simulink model "FDI_sbox_ttime"  (R2018a)
settings: Solver=ode45  StartTime=0.0  StopTime=.4  MaxStep=1e-4  RelTol=1e-3
InitFcn:
  | SimulinkInit
values from neighbouring files (symbols this model uses):
  ssAl = [-2.49999998232 0 0 0 376.789751319 0 -3.33333337039 0 0 376.789751319 0 0 ... (25 elements, 5x5)]    [modeloElectrico.mat]
  ssBl = [24.9999999997 0 0 0 0 0 33.333333333 0 0 0 0 0 ... (15 elements, 5x3)]    [modeloElectrico.mat]
  ssCl = [-0.229841748304 -0.00828937452901 0.991710625471 0 -0.229841748304 0.991710625471 -0.00828937452901 0 0.770158251696 -0.00828937452901 -0.00828937452901 0 ... (20 elements, 4x5)]    [modeloElectrico.mat]
undefined symbols (not defined in the file or in its folder): J, K1, K2, K3, P, Tao1, Tao2
libraries: powerlib x25, truetime x11, dsparch4 x5, mpclib x2, simulink x1, powerlib_meascontrol x1
settings Model: Creator=cmparedes  LastModifiedBy=erich

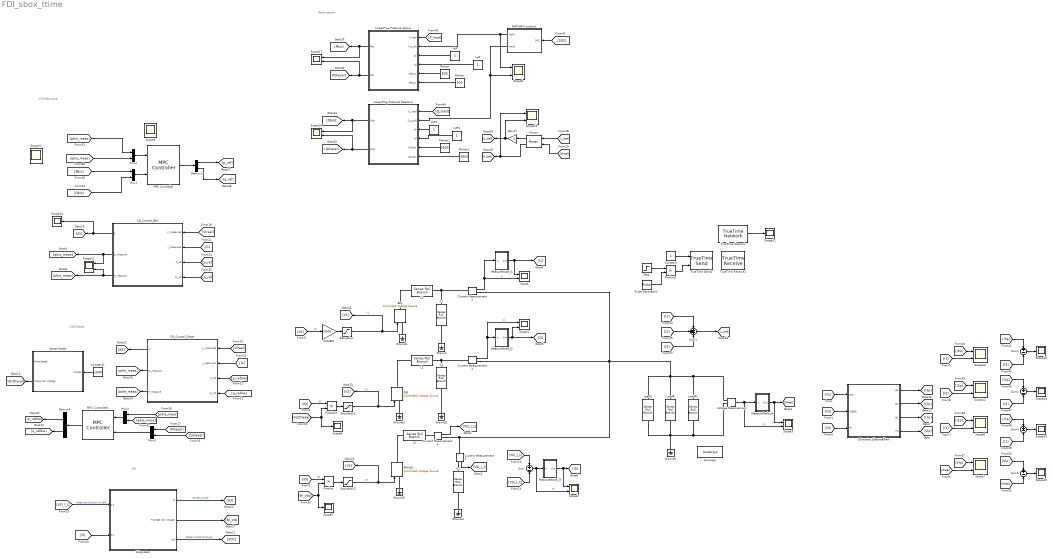
== system FDI_sbox_ttime ==
  note: Optimizacion
  note: CSI2-Diesel
  note: VSI
  note: CSI1-Biomasa
  2VdcBIO : Gain  Gain=2*500
  BIO : powerlib/Electrical Sources/Controlled Voltage Source  Initialize=on  Source_Type=DC  Amplitude=0  Phase=0  Frequency=0  Measurements=None
  C1 : powerlib/Elements/Series RLC Branch  LConnTagsString=__new0  RConnTagsString=__new0  BranchType=C  Resistance=1  Inductance=1e-3  SetiL0=off  InitialCurrent=0  Capacitance=22e-6  Setx0=off  InitialVoltage=0  Measurements=None
  C2 : powerlib/Elements/Series RLC Branch  LConnTagsString=__new0  RConnTagsString=__new0  BranchType=C  Resistance=1  Inductance=1e-3  SetiL0=off  InitialCurrent=0  Capacitance=22e-6  Setx0=off  InitialVoltage=0  Measurements=None
  C3 : powerlib/Elements/Series RLC Branch  LConnTagsString=__new0  RConnTagsString=__new0  BranchType=C  Resistance=1  Inductance=1e-3  SetiL0=off  InitialCurrent=0  Capacitance=610e-6  Setx0=off  InitialVoltage=0  Measurements=None
  CSI_Control_BIO : Subsystem  mask{A=[0.0201   -0.039932     0.01986], B=[1     -1.9966       0.998], T=0.0001, st_time=.1, Dn=[1     -1.0364], Dd=[1    -0.96364]}
      mask prompts: A "Numerador del control PR(z)"; B "Denominador del control PR(z)"; T "Tiempo de muestreo"; st_time "Tiempo_muerto"; Dn "Dn (Numerador de D(z))"; Dd "Dd (numerador de D(z))"
      mask DialogControl descripcion Prompt: Lazo de control de corriente para inversor monofasico. La entrada es un setpoint de potencia [P, Q]. Con ese setpoint se calcula la referencia de corriente sinusoidal deacuerdo a la tension medida de la red. Por lo anterior este controlador solo es valido para un inversor conectado a la red pues hara que se comporte como un CSI.
      mask DialogControl Control2 Prompt: Dn y Dd corresponden al numerador y denominador de la funcion de transferencia en Z (denominada D(z)) que hara un desfase de 90 de las señales medidas de tension y corriente del inversor. Estos desfases permiten mimificar las señales alfa y beta, de esta forma usar la misma teoria de potencia instantanea para el caso monofasico.
  CSI_Control_Diesel : Subsystem  mask{A=[0.0201   -0.039932     0.01986], B=[1     -1.9966       0.998], T=0.0001, st_time=.1, Dn=[1     -1.0364], Dd=[1    -0.96364]}
      mask prompts: A "Numerador del control PR(z)"; B "Denominador del control PR(z)"; T "Tiempo de muestreo"; st_time "Tiempo_muerto"; Dn "Dn (Numerador de D(z))"; Dd "Dd (numerador de D(z))"
      mask DialogControl descripcion Prompt: Lazo de control de corriente para inversor monofasico. La entrada es un setpoint de potencia [P, Q]. Con ese setpoint se calcula la referencia de corriente sinusoidal deacuerdo a la tension medida de la red. Por lo anterior este controlador solo es valido para un inversor conectado a la red pues hara que se comporte como un CSI.
      mask DialogControl Control2 Prompt: Dn y Dd corresponden al numerador y denominador de la funcion de transferencia en Z (denominada D(z)) que hara un desfase de 90 de las señales medidas de tension y corriente del inversor. Estos desfases permiten mimificar las señales alfa y beta, de esta forma usar la misma teoria de potencia instantanea para el caso monofasico.
  Constant : Constant
  Constant1 : Constant  Value=1000
  Current Measurement{1..4} (4 alike) : powerlib/Measurements/Current Measurement  PhasorSimulation=off  OutputType=Complex  PSBequivalent=0
  DIE : powerlib/Electrical Sources/Controlled Voltage Source  Initialize=on  Source_Type=DC  Amplitude=0  Phase=0  Frequency=0  Measurements=None
  Demux1 : Demux  Outputs=2
  Demux4 : Demux  Outputs=2
  Diesel Model : Subsystem
  Gain17 : Gain  Gain=-1
  Ground{,1..6} (7 alike) : powerlib/Elements/Ground  LConnTagsString=a
  L1 : powerlib/Elements/Series RLC Branch  LConnTagsString=__new0  RConnTagsString=__new0  BranchType=RL  Resistance=.1  Inductance=40e-3  SetiL0=off  InitialCurrent=0  Capacitance=1e-6  Setx0=off  InitialVoltage=0  Measurements=None
  L2 : powerlib/Elements/Series RLC Branch  LConnTagsString=__new0  RConnTagsString=__new0  BranchType=RL  Resistance=.1  Inductance=30e-3  SetiL0=off  InitialCurrent=0  Capacitance=1e-6  Setx0=off  InitialVoltage=0  Measurements=None
  L3 : powerlib/Elements/Series RLC Branch  LConnTagsString=__new0  RConnTagsString=__new0  BranchType=RL  Resistance=1e-3  Inductance=5e-3  SetiL0=off  InitialCurrent=0  Capacitance=1e-6  Setx0=off  InitialVoltage=0  Measurements=None
  LinearProg Potencia Activa : MATLAB Function  TreatAsAtomicUnit=on  SystemSampleTime=.03
  LinearProg Potenica Reactiva : MATLAB Function  TreatAsAtomicUnit=on  SystemSampleTime=.03
  LoadC : powerlib/Elements/Series RLC Branch  LConnTagsString=__new0  RConnTagsString=__new0  BranchType=C  Resistance=1  Inductance=1e-3  SetiL0=off  InitialCurrent=0  Capacitance=2000e-6  Setx0=off  InitialVoltage=0  Measurements=None
  LoadR : powerlib/Elements/Series RLC Branch  LConnTagsString=__new0  RConnTagsString=__new0  BranchType=R  Resistance=10  Inductance=1e-3  SetiL0=off  InitialCurrent=0  Capacitance=1e-6  Setx0=off  InitialVoltage=0  Measurements=None
  LoadRL : powerlib/Elements/Series RLC Branch  LConnTagsString=__new0  RConnTagsString=__new0  BranchType=RL  Resistance=10  Inductance=5.2  SetiL0=off  InitialCurrent=0  Capacitance=1e-6  Setx0=off  InitialVoltage=0  Measurements=None
  MATLAB Function1 : MATLAB Function  TreatAsAtomicUnit=on
  MPC Controller : mpclib/MPC Controller  mpcobj=mpcobj  x0=[]  is_multiple=0  enable_value=0  return_u0=off  updateMPCinCallerWorkspace=on  ref_from_ws=off  ref_signal_name=[]  ref_preview=on  md_from_ws=off  md_signal_name=[]  md_preview=on  from_project=off  project_file=MPCtask.mat  md_inport=off  mv_inport=off  cost_outport=off  return_sequence=off  return_qpstatus=off  return_state=off  state_inport=off  lims_inport=off  cc_inport=off  ywt_inport=off  is_designfromscratch=0  uwt_inport=off  duwt_inport=off  rhoeps_inport=off  uref_inport=off  n_ts=0.1  n_p=100  n_mv=2  n_md=0  n_ud=0  n_mo=2  n_uo=0  BlockDataType=double  SampleTimeInherited=off  switch_inport=off
  MPC Controller1 : mpclib/MPC Controller  mpcobj=mpcobj  x0=[]  is_multiple=0  enable_value=0  return_u0=off  updateMPCinCallerWorkspace=on  ref_from_ws=off  ref_signal_name=[]  ref_preview=on  md_from_ws=off  md_signal_name=[]  md_preview=on  from_project=off  project_file=MPCtask.mat  md_inport=off  mv_inport=off  cost_outport=off  return_sequence=off  return_qpstatus=off  return_state=off  state_inport=off  lims_inport=off  cc_inport=off  ywt_inport=off  is_designfromscratch=0  uwt_inport=off  duwt_inport=off  rhoeps_inport=off  uref_inport=off  n_ts=0.1  n_p=100  n_mv=2  n_md=0  n_ud=0  n_mo=2  n_uo=0  BlockDataType=double  SampleTimeInherited=off  switch_inport=off
  MeasureNode_I1 : Subsystem
  MeasureNode_I2 : Subsystem
  MeasureNode_I3 : Subsystem
  MeasureNode_I4 : Subsystem
  Mux{1..4} (4 alike) : Mux  Inputs=2
  PH(VSI) : powerlib/Electrical Sources/Controlled Voltage Source  Initialize=on  Source_Type=DC  Amplitude=0  Phase=0  Frequency=0  Measurements=None
  Pbmax : Constant  Value=500
  Pbmax1 : Constant  Value=3500
  Pdmax : Constant  Value=500
  Pdmax1 : Constant  Value=3500
  Power : powerlib_meascontrol/Measurements/Power  Freq=60  Vinit=[1, 0]  Iinit=[1, 0]  Ts=0
      settings: SourceProductName=Simscape Power Systems
  Product : Product
  Product1 : Product
  Product2 : Product
  Pulse Generator1 : DiscretePulseGenerator  PulseType=Time based  Period=1e-4  PulseWidth=5
  SSversion_ElectricalPart : Subsystem
  Saturation : Saturate  UpperLimit=500  LowerLimit=-500
  Saturation1 : Saturate  UpperLimit=500  LowerLimit=-500
  Saturation2 : Saturate  UpperLimit=500  LowerLimit=-500
  Scope{,1..3,6..13,16..17,21} (15 alike) : Scope  NumInputPorts=2
  Scope{4..5,14..15,18..20,22} (8 alike) : Scope
  Step : Step  Time=5  SampleTime=0
  Subsystem : Subsystem
  Sum{,2..5} (5 alike) : Sum  Inputs=+-
  Sum1 : Sum  Inputs=+++
  TrueTime Network : truetime/TrueTime Network  nwtype=CSMA/CD (Ethernet)  nwnbr=1  nnodes=10  rate=100000000000  minsize=512  lossprob=0  seed=0  bandwidths=[0.5 0.5]  slotsize=512  schedule=[1 1 2]  memsize=80000  buftype=Common buffer  overflow=Retransmit  dynSchedule=0  miniSlotSize=0  NIT=0  QSortMode=FIFO  sync=0  irtSchedule=0  nrtLength=0  nodeGraph=0  scheduleoutput=on
  TrueTime Receive1 : truetime/TrueTime Receive  nwnbr=1  receiver=10  outdim=1  triggeroutput=on  senderoutput=off  lengthoutput=off  priorityoutput=off  timestampoutput=off  signalpoweroutput=off  msgIDoutput=off
  TrueTime Send1 : truetime/TrueTime Send  trigger=falling  nwnbr=1  sender=9  indim=1  recsource=internal  receiver=10  lengthsource=internal  length=70000000  priosource=internal  prio=1  msgIDsource=internal  msgID=0  dynamicSegment=dynamic
  Voltage Measurement : powerlib/Measurements/Voltage Measurement  PhasorSimulation=off  OutputType=Complex  PSBequivalent=0
  kbP : Constant
  kbP1 : Constant
  kdP : Constant
  kdP1 : Constant
  powergui : powerlib/powergui  Priority=1  SimulationMode=Continuous  SampleTime=50e-6  frequency=60  Iterations=50  frequencyindice=0  Pbase=100e6  ErrMax=1e-4  UnitsV=kV  UnitsW=MW  buscounter=0  FunctionMessages=off  echomessages=off  EnableUseOfTLC=off  CurrentSourceSwitches=off  DisableSnubberDevices=off  DisableRonSwitches=off  DisableVfSwitches=off  DisplayEquations=off  SolverType=Tustin/Backward Euler (TBE)  Interpol=off  ExternalGateDelay=off  methode=off  Ts=100  x0status=blocks  SPID=on  SwTol=0  HookPort=off  RestoreLinks=warning  ResistiveCurrentMeasurement=off  Frange=[0:2:500]  Ylog=off  Xlog=on  ShowGrid=off  save=off  variable=ZData  structure=0  ZoomFFT=off  StartTime=0.0  cycles=1  DisplayStyle=1  fundamental=60  FreqAxis=off  MaxFrequency=1000  frequencyindicesteady=1  RmsSteady=1  display=off
  wires:
  [d1] -> 2VdcBIO/1  "d1"
  [d2] -> Product1/1  "d2"
  [d3] -> Product/1  "d3"
  Current Measurement2/1 -> MeasureNode_I1/1(in), Scope/2  "I1"
  Current Measurement1/1 -> Scope1/1, MeasureNode_I2/1(in)  "I2"
  Sum/1 -> MeasureNode_I3/1(in), Scope2/2  "I3"
  Voltage Measurement/1 -> Scope3/2, MeasureNode_I4/1(in)  "VL"
  Pdmax1/1 -> LinearProg Potenica Reactiva/5(QdMax)
  [Pbio] -> Mux1/1
  Mux1/1 -> MPC Controller/2
  [SOC] -> MATLAB Function1/1(SOC)
  [Qbio] -> Mux1/2
  [Qdiesel] -> Mux3/2
  [qdie_meas] -> Mux4/2
  [p_refdie] -> CSI_Control_Diesel/3(P_ref)
  [Pdiesel] -> Mux3/1
  [Q_load] -> LinearProg Potenica Reactiva/1(Q_load)
  CSI_Control_BIO/2(Q_measure) -> [qbio_meas], Scope21/1
  [qbio_meas] -> Mux2/2
  Pbmax1/1 -> LinearProg Potenica Reactiva/6(QbMax)
  [q_refdie] -> CSI_Control_Diesel/4(Q_ref)
  LinearProg Potencia Activa/1(Pbo) -> Scope17/1, [Pbio]
  kdP1/1 -> LinearProg Potenica Reactiva/4(kd)
  MATLAB Function1/2(MaxQ) -> Scope9/2, LinearProg Potenica Reactiva/2(Q_e_alt)
  CSI_Control_BIO/1(D) -> [d1], Scope14/1
  Demux1/2 -> [q_ref]
  Pdmax/1 -> LinearProg Potencia Activa/5(PdMax)
  Pbmax/1 -> LinearProg Potencia Activa/6(PbMax)
  [P_load] -> LinearProg Potencia Activa/1(P_load)
  Demux4/2 -> [q_refdie]
  kbP/1 -> LinearProg Potencia Activa/3(kb)
  Mux4/1 -> MPC Controller1/1
  Demux1/1 -> [p_ref]
  kbP1/1 -> LinearProg Potenica Reactiva/3(kb)
  LinearProg Potenica Reactiva/1(Qbo) -> Scope16/1, [Qbio]
  MPC Controller/1 -> Demux1/1
  [pdie_meas] -> Mux4/1
  LinearProg Potenica Reactiva/2(Qdo) -> Scope16/2, [Qdiesel]
  Mux3/1 -> MPC Controller1/2
  Demux4/1 -> [p_refdie]
  CSI_Control_Diesel/2(Q_measure) -> [qdie_meas]
  Mux2/1 -> MPC Controller/1
  [q_ref] -> CSI_Control_BIO/4(Q_ref)
  CSI_Control_BIO/3(P_measure) -> Scope21/2, [pbio_meas]
  CSI_Control_Diesel/3(P_measure) -> [pdie_meas]
  [Vlreal] -> CSI_Control_BIO/1(V_measured)
  MPC Controller1/1 -> Demux4/1
  LinearProg Potencia Activa/2(Pdo) -> Scope17/2, [Pdiesel]
  MATLAB Function1/1(MaxP) -> Scope9/1, LinearProg Potencia Activa/2(P_e_alt)
  kdP/1 -> LinearProg Potencia Activa/4(kd)
  [p_ref] -> CSI_Control_BIO/3(P_ref)
  2VdcBIO/1 -> Saturation/1
  Saturation/1 -> [V1], BIO/1  "V1"
  Product1/1 -> Saturation1/1
  Product/1 -> Saturation2/1
  Saturation1/1 -> [V2], DIE/1  "V2"
  Saturation2/1 -> [V3], PH(VSI)/1  "V3"
  [V1] -> SSversion_ElectricalPart/1(BIO)
  [V2] -> SSversion_ElectricalPart/2(DIESEL)
  [V3] -> SSversion_ElectricalPart/3(PV)
  SSversion_ElectricalPart/1(Ip3) -> [I3p]
  SSversion_ElectricalPart/2(Ip2) -> [I2p]
  SSversion_ElectricalPart/3(Ip1) -> [I1p]
  Current Measurement4/1 -> [VSI_I_L]
  Current Measurement3/1 -> [VSI_I_C]
  [VSI_I_L] -> Sum/1
  [VSI_I_C] -> Sum/2
  [VSI_I_L] -> Subsystem/1(IL3)  "measured inductor current"
  Subsystem/1(D) -> [d3]  "VSI duty Cycle"
  Subsystem/2(H bridge Vdc Voltage) -> [Br_Vdc]
  Subsystem/3(soc) -> [SOC]  "battery state of charge"
  Constant1/1 -> Diesel Model/1(Caudal)
  Diesel Model/2(Output DC Voltage) -> [VdcDiesel]
  CSI_Control_Diesel/1(D) -> [d2]
  [Vlreal] -> CSI_Control_Diesel/1(V_measured)
  [VdcDiesel] -> Scope4/1, Product1/2
  [I1] -> CSI_Control_BIO/2(I_measured)
  [I2] -> CSI_Control_Diesel/2(I_measured)
  [I2] -> Sum1/2
  [I1] -> Sum1/1
  [I3] -> Sum1/3
  Sum1/1 -> [I_Load]
  [I_Load] -> Power/2
  [Vlreal] -> Power/1
  [Br_Vdc] -> Product/2, Scope5/1
  [I3] -> Subsystem/2(IL1)
  SSversion_ElectricalPart/4(Vlp) -> [Vlp]
  [Vlreal] -> Scope7/2
  [pbio_meas] -> Mux2/1
  Power/2 -> Gain17/1
  Gain17/1 -> [Q_load], Scope10/2
  Power/1 -> [P_load], Scope10/1
  MeasureNode_I1/1(Out) -> [I1], Scope/1
  MeasureNode_I2/1(Out) -> [I2], Scope1/2
  MeasureNode_I3/1(Out) -> Scope2/1, [I3]
  MeasureNode_I4/1(Out) -> [Vlreal], Scope3/1
  [Vlp] -> Scope7/1
  [I1p] -> Scope8/1
  [I1] -> Scope8/2
  [I2] -> Scope12/2
  [I2p] -> Scope12/1
  [I3] -> Scope13/2
  [I3p] -> Scope13/1
  Sum2/1 -> Scope15/1
  [I3p] -> Sum2/1
  [I3] -> Sum2/2
  [I2] -> Sum3/2
  [I2p] -> Sum3/1
  Sum3/1 -> Scope18/1
  Sum4/1 -> Scope19/1
  [I1p] -> Sum4/1
  [I1] -> Sum4/2
  [Vlreal] -> Sum5/2
  [Vlp] -> Sum5/1
  Sum5/1 -> Scope20/1
  TrueTime Network/1 -> Scope22/1
  Constant/1 -> TrueTime Send1/1
  Product2/1 -> TrueTime Send1/2
  Step/1 -> Product2/1
  Pulse Generator1/1 -> Product2/2
  connections:
  L1/LConn1 -- BIO/RConn1
  Ground/LConn1 -- C1/RConn1
  Ground1/LConn1 -- BIO/LConn1
  Ground2/LConn1 -- C2/RConn1
  Ground3/LConn1 -- DIE/LConn1
  L2/LConn1 -- DIE/RConn1
  L3/LConn1 -- PH(VSI)/RConn1
  Ground5/LConn1 -- PH(VSI)/LConn1
  Ground4/LConn1 -- C3/RConn1
  Ground6/LConn1 -- Voltage Measurement/LConn2 -- LoadRL/RConn1 -- LoadC/RConn1 -- LoadR/RConn1
  LoadC/LConn1 -- Current Measurement3/LConn1 -- Current Measurement4/RConn1 -- Current Measurement2/RConn1 -- Current Measurement1/RConn1 -- LoadR/LConn1 -- LoadRL/LConn1 -- Voltage Measurement/LConn1
  L2/RConn1 -- Current Measurement1/LConn1 -- C2/LConn1
  L1/RConn1 -- Current Measurement2/LConn1 -- C1/LConn1
  Current Measurement3/RConn1 -- C3/LConn1
  Current Measurement4/LConn1 -- L3/RConn1

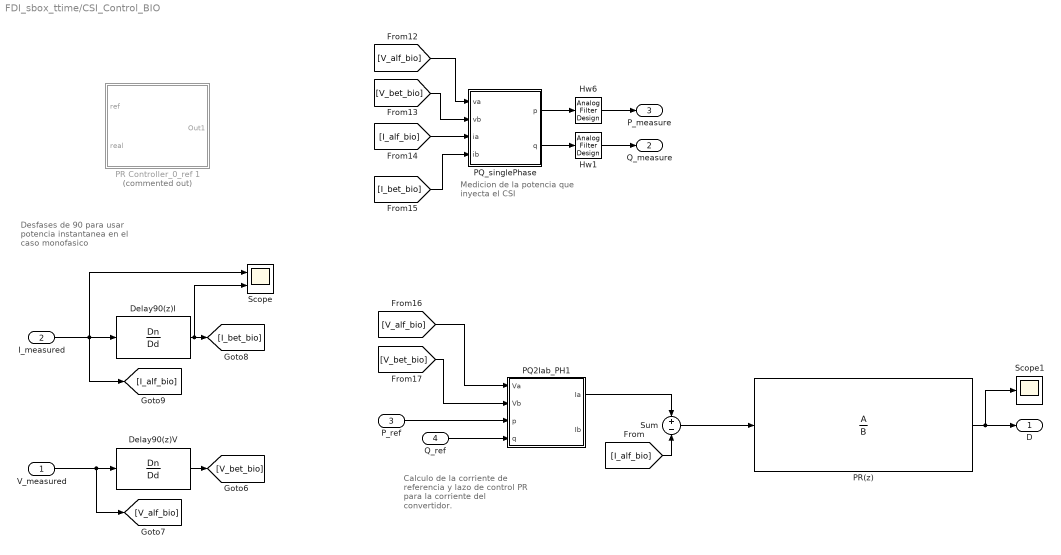
== system FDI_sbox_ttime/CSI_Control_BIO ==
  note: Medicion de la potencia que inyecta el CSI
  note: Desfases de 90 para usar potencia
      | instantanea en el caso monofasico
  note: Calculo de la corriente de referencia
      | y lazo de control PR para la corriente
      | del convertidor.
  V_measured : Inport
  I_measured : Inport  Port=2
  P_ref : Inport  Port=3
  Q_ref : Inport  Port=4
  Delay90(z)I : DiscreteTransferFcn  Numerator=Dn  Denominator=Dd  SampleTime=T
  Delay90(z)V : DiscreteTransferFcn  Numerator=Dn  Denominator=Dd  SampleTime=T
  Hw1 : dsparch4/Analog Filter Design  method=Bessel  filttype=Lowpass  N=4  Wlo=30*2*pi  Whi=80  Rp=2  Rs=80
  Hw6 : dsparch4/Analog Filter Design  method=Bessel  filttype=Lowpass  N=4  Wlo=30*2*pi  Whi=80  Rp=2  Rs=80
  PQ2Iab_PH1 : MATLAB Function  TreatAsAtomicUnit=on
  PQ_singlePhase : MATLAB Function  TreatAsAtomicUnit=on
  PR Controller_0_ref 1 : Subsystem  Commented=on  mask{Kp=40/100, Ki=200, wa=2, w0=60*2*pi, st_time=1e-3}
      mask prompts: Kp "Ganancia Proporcional"; Ki "Ganancia Integral"; wa "Ancho camapana resonancia"; w0 "Frecuencia Central"; st_time "Tiempo muerto (Start)"
      mask Display:
      | port_label('input',1,'ref')
      | port_label('input',2,'sens')
      | port_label('output',1,'out')
      | 
      | plot(.4+[0:.01:pi/10], .32+sin(40*[0:.01:pi/10])/13)
      | 
      | plot([.4 .6],.05+[.5 .7])
      | plot([.4 .6],.05+[.9 .7])
      | plot([.4 .4],.05+[.9 .5])
      | 
      | text(.27,.37,'\fontsize{25} \int', 'texmode', 'on')
  PR(z) : DiscreteTransferFcn  Numerator=A  Denominator=B  SampleTime=T
  Scope : Scope  NumInputPorts=2
  Scope1 : Scope
  Sum : Sum  Inputs=+-
  D : Outport
  Q_measure : Outport  Port=2
  P_measure : Outport  Port=3
  wires:
  I_measured/1 -> Scope/1, Delay90(z)I/1, [I_alf_bio]
  PQ_singlePhase/2(q) -> Hw1/1
  [V_bet_bio] -> PQ2Iab_PH1/2(Vb)
  Delay90(z)I/1 -> Scope/2, [I_bet_bio]
  [I_bet_bio] -> PQ_singlePhase/4(ib)
  [I_alf_bio] -> PQ_singlePhase/3(ia)
  [V_alf_bio] -> PQ2Iab_PH1/1(Va)
  PQ_singlePhase/1(p) -> Hw6/1
  Delay90(z)V/1 -> [V_bet_bio]
  [V_bet_bio] -> PQ_singlePhase/2(vb)
  [V_alf_bio] -> PQ_singlePhase/1(va)
  V_measured/1 -> Delay90(z)V/1, [V_alf_bio]
  P_ref/1 -> PQ2Iab_PH1/3(p)
  Q_ref/1 -> PQ2Iab_PH1/4(q)
  Sum/1 -> PR(z)/1
  [I_alf_bio] -> Sum/2
  PQ2Iab_PH1/1(Ia) -> Sum/1
  PR(z)/1 -> Scope1/1, D/1
  Hw6/1 -> P_measure/1
  Hw1/1 -> Q_measure/1

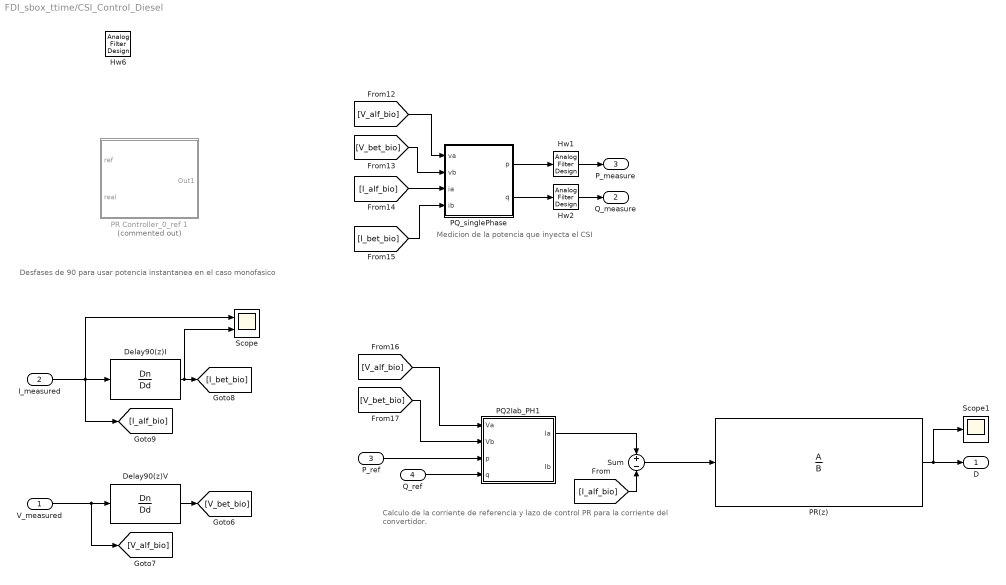
== system FDI_sbox_ttime/CSI_Control_Diesel ==
  note: Medicion de la potencia que inyecta el CSI
  note: Desfases de 90 para usar potencia
      | instantanea en el caso monofasico
  note: Calculo de la corriente de referencia
      | y lazo de control PR para la corriente
      | del convertidor.
  V_measured : Inport
  I_measured : Inport  Port=2
  P_ref : Inport  Port=3
  Q_ref : Inport  Port=4
  Delay90(z)I : DiscreteTransferFcn  Numerator=Dn  Denominator=Dd  SampleTime=T
  Delay90(z)V : DiscreteTransferFcn  Numerator=Dn  Denominator=Dd  SampleTime=T
  Hw1 : dsparch4/Analog Filter Design  method=Bessel  filttype=Lowpass  N=4  Wlo=30*2*pi  Whi=80  Rp=2  Rs=80
  Hw2 : dsparch4/Analog Filter Design  method=Bessel  filttype=Lowpass  N=4  Wlo=30*2*pi  Whi=80  Rp=2  Rs=80
  Hw6 : dsparch4/Analog Filter Design  method=Bessel  filttype=Lowpass  N=4  Wlo=30*2*pi  Whi=80  Rp=2  Rs=80
  PQ2Iab_PH1 : MATLAB Function  TreatAsAtomicUnit=on
  PQ_singlePhase : MATLAB Function  TreatAsAtomicUnit=on
  PR Controller_0_ref 1 : Subsystem  Commented=on  mask{Kp=40/100, Ki=200, wa=2, w0=60*2*pi, st_time=1e-3}
      mask prompts: Kp "Ganancia Proporcional"; Ki "Ganancia Integral"; wa "Ancho camapana resonancia"; w0 "Frecuencia Central"; st_time "Tiempo muerto (Start)"
      mask Display:
      | port_label('input',1,'ref')
      | port_label('input',2,'sens')
      | port_label('output',1,'out')
      | 
      | plot(.4+[0:.01:pi/10], .32+sin(40*[0:.01:pi/10])/13)
      | 
      | plot([.4 .6],.05+[.5 .7])
      | plot([.4 .6],.05+[.9 .7])
      | plot([.4 .4],.05+[.9 .5])
      | 
      | text(.27,.37,'\fontsize{25} \int', 'texmode', 'on')
  PR(z) : DiscreteTransferFcn  Numerator=A  Denominator=B  SampleTime=T
  Scope : Scope  NumInputPorts=2
  Scope1 : Scope
  Sum : Sum  Inputs=+-
  D : Outport
  Q_measure : Outport  Port=2
  P_measure : Outport  Port=3
  wires:
  I_measured/1 -> Scope/1, Delay90(z)I/1, [I_alf_bio]
  PQ_singlePhase/2(q) -> Hw2/1
  [V_bet_bio] -> PQ2Iab_PH1/2(Vb)
  Delay90(z)I/1 -> Scope/2, [I_bet_bio]
  [I_bet_bio] -> PQ_singlePhase/4(ib)
  [I_alf_bio] -> PQ_singlePhase/3(ia)
  [V_alf_bio] -> PQ2Iab_PH1/1(Va)
  PQ_singlePhase/1(p) -> Hw1/1
  Delay90(z)V/1 -> [V_bet_bio]
  [V_bet_bio] -> PQ_singlePhase/2(vb)
  [V_alf_bio] -> PQ_singlePhase/1(va)
  V_measured/1 -> Delay90(z)V/1, [V_alf_bio]
  P_ref/1 -> PQ2Iab_PH1/3(p)
  Q_ref/1 -> PQ2Iab_PH1/4(q)
  Sum/1 -> PR(z)/1
  [I_alf_bio] -> Sum/2
  PQ2Iab_PH1/1(Ia) -> Sum/1
  PR(z)/1 -> Scope1/1, D/1
  Hw1/1 -> P_measure/1
  Hw2/1 -> Q_measure/1

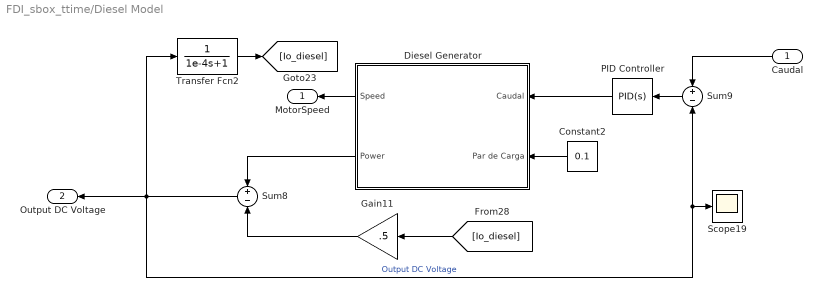
== system FDI_sbox_ttime/Diesel Model ==
  Caudal : Inport
  Constant2 : Constant  Value=0.1
  Diesel Generator : Subsystem
  Gain11 : Gain  Gain=.5
  PID Controller : simulink/Continuous/PID Controller  Controller=PID  TimeDomain=Continuous-time  SampleTime=-1  IntegratorMethod=Forward Euler  FilterMethod=Forward Euler  Form=Parallel  UseFilter=on  ControllerParametersSource=internal  P=0.000853612192208084  I=3.94394231511782e-05  D=0.00224356290205903  N=0.155980576752107  InitialConditionSource=internal  InitialConditionForIntegrator=0  InitialConditionForFilter=0  ExternalReset=none  LimitOutput=off  UpperSaturationLimit=inf  LowerSaturationLimit=-inf  LinearizeAsGain=on  AntiWindupMode=none  Kb=1  TrackingMode=off  Kt=1  PParamMin=[]  PParamMax=[]  IParamMin=[]  IParamMax=[]  DParamMin=[]  DParamMax=[]  NParamMin=[]  NParamMax=[]  KbParamMin=[]  KbParamMax=[]  KtParamMin=[]  KtParamMax=[]  POutMin=[]  POutMax=[]  IOutMin=[]  IOutMax=[]  DOutMin=[]  DOutMax=[]  NOutMin=[]  NOutMax=[]  KbOutMin=[]  KbOutMax=[]  KtOutMin=[]  KtOutMax=[]  IntegratorOutMin=[]  IntegratorOutMax=[]  FilterOutMin=[]  FilterOutMax=[]  SumOutMin=[]  SumOutMax=[]  SumI1OutMin=[]  SumI1OutMax=[]  SumI2OutMin=[]  SumI2OutMax=[]  SumI3OutMin=[]  SumI3OutMax=[]  SumDOutMin=[]  SumDOutMax=[]  SaturationOutMin=[]  SaturationOutMax=[]  IntegratorContinuousStateAttributes=''  IntegratorStateMustResolveToSignalObject=off  IntegratorRTWStateStorageClass=Auto  FilterContinuousStateAttributes=''  FilterStateMustResolveToSignalObject=off  FilterRTWStateStorageClass=Auto  DifferentiatorICPrevScaledInput=0  DifferentiatorOutMin=[]  DifferentiatorOutMax=[]  InitialConditionSetting=State (most efficient)  FilterDiffOutCoefMin=[]  FilterDiffOutCoefMax=[]  SumDenOutMin=[]  SumDenOutMax=[]  SumNumOutMin=[]  SumNumOutMax=[]  ReciprocalOutMin=[]  ReciprocalOutMax=[]  DivideOutMin=[]  DivideOutMax=[]  TunerSelectOption=Transfer Function Based (PID Tuner App)
  Scope19 : Scope
  Sum8 : Sum  Inputs=+-
  Sum9 : Sum  Inputs=+-
  Transfer Fcn2 : TransferFcn  Denominator=[1e-4 1]
  MotorSpeed : Outport
  Output DC Voltage : Outport  Port=2
  wires:
  Transfer Fcn2/1 -> [Io_diesel]
  Sum8/1 -> Output DC Voltage/1, Scope19/1, Sum9/2, Transfer Fcn2/1  "Output DC Voltage"
  Constant2/1 -> Diesel Generator/2(Par de Carga)
  PID Controller/1 -> Diesel Generator/1(Caudal)
  Gain11/1 -> Sum8/2
  Diesel Generator/2(Power) -> Sum8/1
  [Io_diesel] -> Gain11/1
  Caudal/1 -> Sum9/1
  Sum9/1 -> PID Controller/1
  Diesel Generator/1(Speed) -> MotorSpeed/1

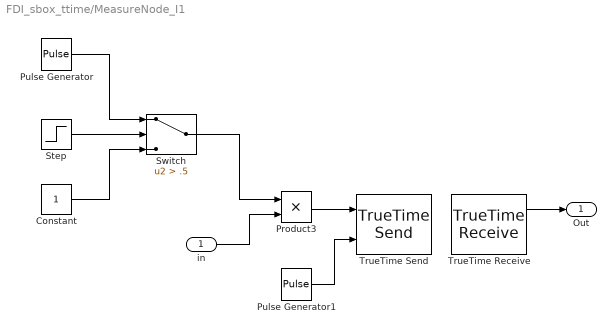
== system FDI_sbox_ttime/MeasureNode_I1 ==
  in : Inport
  Constant : Constant
  Product3 : Product
  Pulse Generator : DiscretePulseGenerator  PulseType=Time based  Period=50e-3  PulseWidth=50
  Pulse Generator1 : DiscretePulseGenerator  PulseType=Time based  Period=1e-4  PulseWidth=50
  Step : Step  SampleTime=0
  Switch : Switch  Criteria=u2 > Threshold  Threshold=.5
  TrueTime Receive : truetime/TrueTime Receive  nwnbr=1  receiver=2  outdim=1  triggeroutput=on  senderoutput=off  lengthoutput=off  priorityoutput=off  timestampoutput=off  signalpoweroutput=off  msgIDoutput=off
  TrueTime Send : truetime/TrueTime Send  trigger=falling  nwnbr=1  sender=1  indim=1  recsource=internal  receiver=2  lengthsource=internal  length=1000  priosource=internal  prio=1  msgIDsource=internal  msgID=0  dynamicSegment=dynamic
  Out : Outport
  wires:
  Pulse Generator/1 -> Switch/1
  Constant/1 -> Switch/3
  Switch/1 -> Product3/1
  Step/1 -> Switch/2
  in/1 -> Product3/2
  Pulse Generator1/1 -> TrueTime Send/2
  Product3/1 -> TrueTime Send/1
  TrueTime Receive/1 -> Out/1

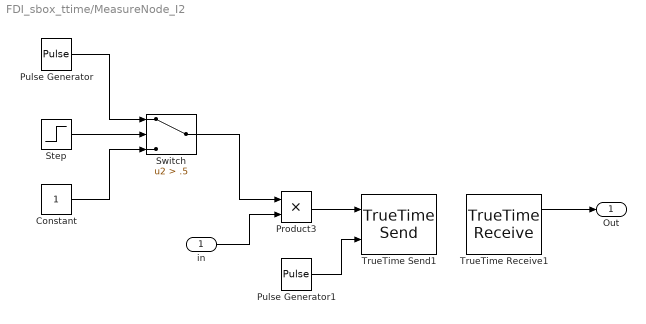
== system FDI_sbox_ttime/MeasureNode_I2 ==
  in : Inport
  Constant : Constant
  Product3 : Product
  Pulse Generator : DiscretePulseGenerator  PulseType=Time based  Period=50e-3  PulseWidth=50
  Pulse Generator1 : DiscretePulseGenerator  PulseType=Time based  Period=1e-4  PulseWidth=30
  Step : Step  Time=.2  SampleTime=0
  Switch : Switch  Criteria=u2 > Threshold  Threshold=.5
  TrueTime Receive1 : truetime/TrueTime Receive  nwnbr=1  receiver=4  outdim=1  triggeroutput=on  senderoutput=off  lengthoutput=off  priorityoutput=off  timestampoutput=off  signalpoweroutput=off  msgIDoutput=off
  TrueTime Send1 : truetime/TrueTime Send  trigger=falling  nwnbr=1  sender=3  indim=1  recsource=internal  receiver=4  lengthsource=internal  length=1000  priosource=internal  prio=1  msgIDsource=internal  msgID=0  dynamicSegment=dynamic
  Out : Outport
  wires:
  in/1 -> Product3/2
  Step/1 -> Switch/2
  Switch/1 -> Product3/1
  Constant/1 -> Switch/3
  Pulse Generator/1 -> Switch/1
  Pulse Generator1/1 -> TrueTime Send1/2
  Product3/1 -> TrueTime Send1/1
  TrueTime Receive1/1 -> Out/1

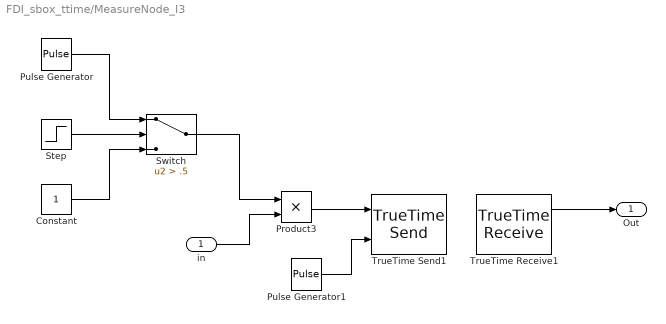
== system FDI_sbox_ttime/MeasureNode_I3 ==
  in : Inport
  Constant : Constant
  Product3 : Product
  Pulse Generator : DiscretePulseGenerator  PulseType=Time based  Period=50e-3  PulseWidth=50
  Pulse Generator1 : DiscretePulseGenerator  PulseType=Time based  Period=1e-4  PulseWidth=5
  Step : Step  Time=5  SampleTime=0
  Switch : Switch  Criteria=u2 > Threshold  Threshold=.5
  TrueTime Receive1 : truetime/TrueTime Receive  nwnbr=1  receiver=6  outdim=1  triggeroutput=on  senderoutput=off  lengthoutput=off  priorityoutput=off  timestampoutput=off  signalpoweroutput=off  msgIDoutput=off
  TrueTime Send1 : truetime/TrueTime Send  trigger=falling  nwnbr=1  sender=5  indim=1  recsource=internal  receiver=6  lengthsource=internal  length=1000  priosource=internal  prio=1  msgIDsource=internal  msgID=0  dynamicSegment=dynamic
  Out : Outport
  wires:
  Pulse Generator/1 -> Switch/1
  Constant/1 -> Switch/3
  Switch/1 -> Product3/1
  Step/1 -> Switch/2
  in/1 -> Product3/2
  Pulse Generator1/1 -> TrueTime Send1/2
  Product3/1 -> TrueTime Send1/1
  TrueTime Receive1/1 -> Out/1

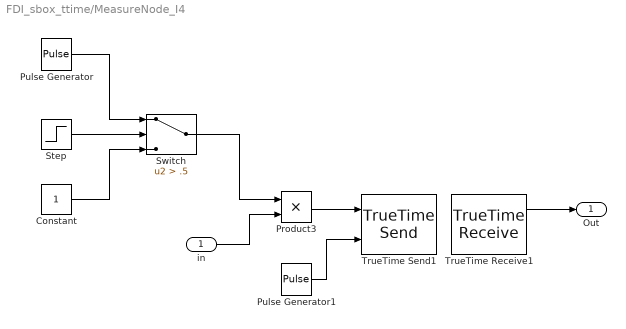
== system FDI_sbox_ttime/MeasureNode_I4 ==
  in : Inport
  Constant : Constant
  Product3 : Product
  Pulse Generator : DiscretePulseGenerator  PulseType=Time based  Period=50e-3  PulseWidth=50
  Pulse Generator1 : DiscretePulseGenerator  PulseType=Time based  Period=1e-4  PulseWidth=5  PhaseDelay=10e-3
  Step : Step  Time=5  SampleTime=0
  Switch : Switch  Criteria=u2 > Threshold  Threshold=.5
  TrueTime Receive1 : truetime/TrueTime Receive  nwnbr=1  receiver=8  outdim=1  triggeroutput=on  senderoutput=off  lengthoutput=off  priorityoutput=off  timestampoutput=off  signalpoweroutput=off  msgIDoutput=off
  TrueTime Send1 : truetime/TrueTime Send  trigger=falling  nwnbr=1  sender=7  indim=1  recsource=internal  receiver=8  lengthsource=internal  length=1000  priosource=internal  prio=1  msgIDsource=internal  msgID=0  dynamicSegment=dynamic
  Out : Outport
  wires:
  in/1 -> Product3/2
  Step/1 -> Switch/2
  Switch/1 -> Product3/1
  Constant/1 -> Switch/3
  Pulse Generator/1 -> Switch/1
  Pulse Generator1/1 -> TrueTime Send1/2
  Product3/1 -> TrueTime Send1/1
  TrueTime Receive1/1 -> Out/1

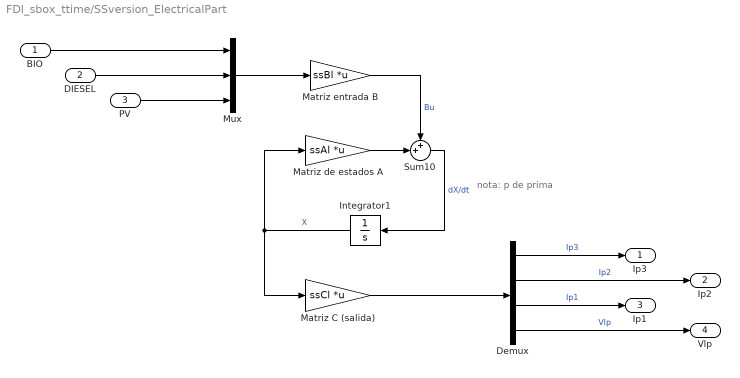
== system FDI_sbox_ttime/SSversion_ElectricalPart ==
  note: nota: p de prima
  BIO : Inport
  DIESEL : Inport  Port=2
  PV : Inport  Port=3
  Demux : Demux
  Integrator1 : Integrator
  Matriz C (salida) : Gain  Gain=ssCl  Multiplication=Matrix(K*u)
  Matriz de estados A : Gain  Gain=ssAl  Multiplication=Matrix(K*u)
  Matriz entrada B : Gain  Gain=ssBl  Multiplication=Matrix(K*u)
  Mux : Mux  Inputs=3
  Sum10 : Sum  Inputs=++|
  Ip3 : Outport
  Ip2 : Outport  Port=2
  Ip1 : Outport  Port=3
  Vlp : Outport  Port=4
  wires:
  Matriz entrada B/1 -> Sum10/1  "Bu"
  Matriz de estados A/1 -> Sum10/2
  Demux/1 -> Ip3/1  "Ip3"
  Integrator1/1 -> Matriz C (salida)/1, Matriz de estados A/1  "X"
  Demux/4 -> Vlp/1  "Vlp"
  Demux/2 -> Ip2/1  "Ip2"
  Sum10/1 -> Integrator1/1  "dX/dt"
  Mux/1 -> Matriz entrada B/1
  PV/1 -> Mux/3
  Demux/3 -> Ip1/1  "Ip1"
  DIESEL/1 -> Mux/2
  BIO/1 -> Mux/1
  Matriz C (salida)/1 -> Demux/1

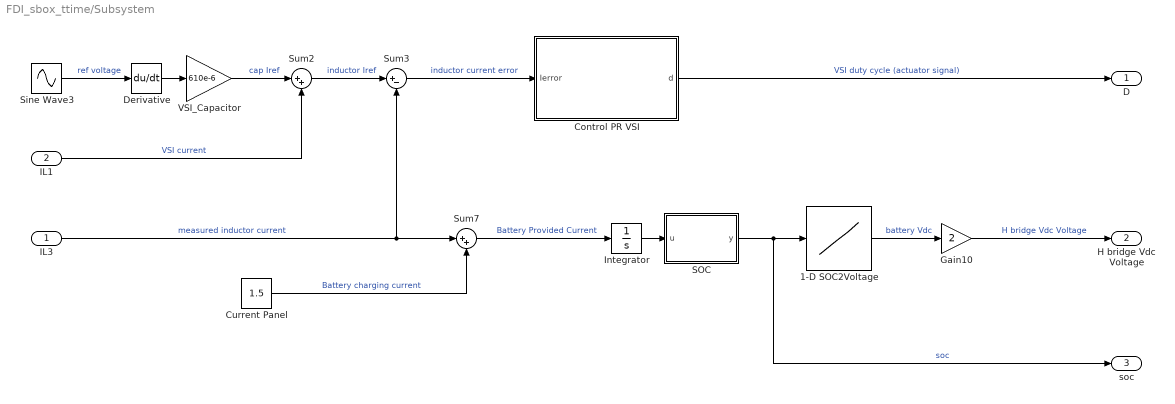
== system FDI_sbox_ttime/Subsystem ==
  IL3 : Inport
  IL1 : Inport  Port=2
  1-D SOC2Voltage : Lookup_n-D  NumberOfTableDimensions=1  BreakpointsForDimension1=[0 10 20 30 40 50 70 80 100]  Table=[0 10 200 500 800 1000 1140 1150 1200]  InternalRulePriority=Speed  RndMeth=Simplest  InputSameDT=on
  Control PR VSI : Subsystem
  Current Panel : Constant  Value=1.5
  Derivative : Derivative
  Gain10 : Gain  Gain=2
  Integrator : Integrator  LimitOutput=on  UpperSaturationLimit=1  LowerSaturationLimit=0
  "SOC " : MATLAB Function  TreatAsAtomicUnit=on
  Sine Wave3 : Sin  Amplitude=170  Frequency=2*pi*60  SampleTime=0
  Sum2 : Sum  Inputs=|++
  Sum3 : Sum  Inputs=|+-
  Sum7 : Sum  Inputs=|++
  VSI_Capacitor : Gain  Gain=610e-6
  D : Outport
  H bridge Vdc Voltage : Outport  Port=2
  soc : Outport  Port=3
  wires:
  Sine Wave3/1 -> Derivative/1  "ref voltage"
  Current Panel/1 -> Sum7/2  "Battery charging current"
  Derivative/1 -> VSI_Capacitor/1
  VSI_Capacitor/1 -> Sum2/1  "cap Iref"
  Sum7/1 -> Integrator/1  "Battery Provided Current"
  Integrator/1 -> "SOC "/1(u)
  1-D SOC2Voltage/1 -> Gain10/1  "battery Vdc"
  Control PR VSI/1(d) -> D/1  "VSI duty cycle (actuator signal)"
  IL3/1 -> Sum7/1, Sum3/2  "measured inductor current"
  "SOC "/1(y) -> soc/1, 1-D SOC2Voltage/1  "soc"
  IL1/1 -> Sum2/2  "VSI current"
  Sum3/1 -> Control PR VSI/1(Ierror)  "inductor current error"
  Gain10/1 -> H bridge Vdc Voltage/1  "H bridge Vdc Voltage"
  Sum2/1 -> Sum3/1  "inductor Iref"

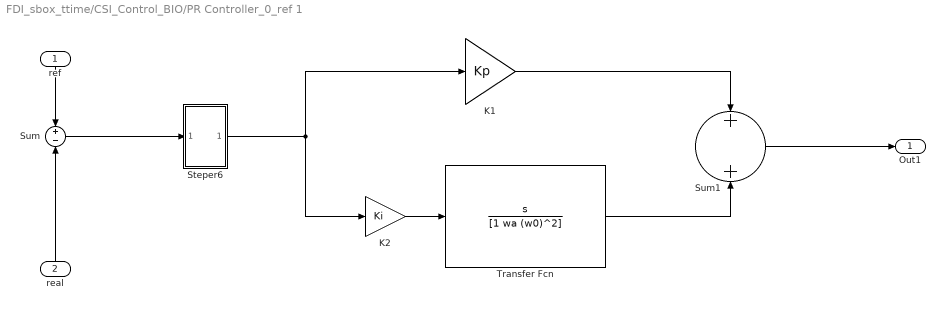
== system FDI_sbox_ttime/CSI_Control_BIO/PR Controller_0_ref 1 ==
  ref : Inport
  real : Inport  Port=2
  K1 : Gain  Gain=Kp
  K2 : Gain  Gain=Ki
  Steper6 : Subsystem
  Sum : Sum  Inputs=+-
  Sum1 : Sum  Inputs=+|+
  Transfer Fcn : TransferFcn  Numerator=[1 0]  Denominator=[1 wa (w0)^2]
  Out1 : Outport
  wires:
  real/1 -> Sum/2
  ref/1 -> Sum/1
  Sum/1 -> Steper6/1(In1)
  K1/1 -> Sum1/1
  Transfer Fcn/1 -> Sum1/2
  K2/1 -> Transfer Fcn/1
  Steper6/1(Out1) -> K1/1, K2/1
  Sum1/1 -> Out1/1

== system FDI_sbox_ttime/CSI_Control_Diesel/PR Controller_0_ref 1 ==
  ref : Inport
  real : Inport  Port=2
  K1 : Gain  Gain=Kp
  K2 : Gain  Gain=Ki
  Steper6 : Subsystem
  Sum : Sum  Inputs=+-
  Sum1 : Sum  Inputs=+|+
  Transfer Fcn : TransferFcn  Numerator=[1 0]  Denominator=[1 wa (w0)^2]
  Out1 : Outport
  wires:
  real/1 -> Sum/2
  ref/1 -> Sum/1
  Sum/1 -> Steper6/1(In1)
  K1/1 -> Sum1/1
  Transfer Fcn/1 -> Sum1/2
  K2/1 -> Transfer Fcn/1
  Steper6/1(Out1) -> K1/1, K2/1
  Sum1/1 -> Out1/1

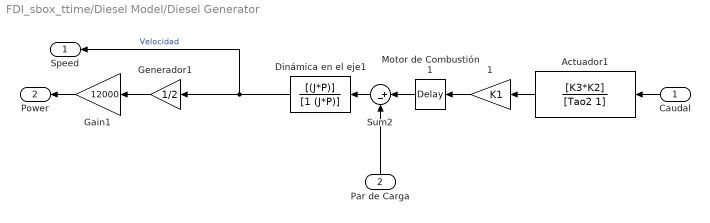
== system FDI_sbox_ttime/Diesel Model/Diesel Generator ==
  Caudal : Inport
  Par de Carga : Inport  Port=2
  " 1" : Gain  Gain=K1
  " Generador1" : Gain  Gain=1/2
  Actuador1 : TransferFcn  Numerator=[K3*K2]  Denominator=[Tao2 1]
  Dinámica en el eje1 : TransferFcn  Numerator=[(J*P)]  Denominator=[1 (J*P)]
  Gain1 : Gain  Gain=12000
  Motor de Combustión1 : TransportDelay  DelayTime=Tao1
  Sum2 : Sum  Inputs=|+-
  Speed : Outport
  Power : Outport  Port=2
  wires:
  " 1"/1 -> Motor de Combustión1/1
  " Generador1"/1 -> Gain1/1
  Motor de Combustión1/1 -> Sum2/1
  Actuador1/1 -> " 1"/1
  Dinámica en el eje1/1 -> Speed/1, " Generador1"/1  "Velocidad"
  Sum2/1 -> Dinámica en el eje1/1
  Caudal/1 -> Actuador1/1
  Par de Carga/1 -> Sum2/2
  Gain1/1 -> Power/1

== system FDI_sbox_ttime/Subsystem/Control PR VSI ==
  Ierror : Inport
  Constant2 : Constant  Value=0
  Gain2 : Gain  Gain=.002
  Sum5 : Sum  Inputs=+|+
  Sum9 : Sum  Inputs=|++
  Transfer Fcn2 : TransferFcn  Numerator=[2 0]  Denominator=[1 2 (2*pi*60)^2]
  d : Outport
  wires:
  Constant2/1 -> Sum9/2
  Sum5/1 -> Sum9/1
  Transfer Fcn2/1 -> Sum5/2
  Gain2/1 -> Sum5/1
  Ierror/1 -> Transfer Fcn2/1, Gain2/1
  Sum9/1 -> d/1

== system FDI_sbox_ttime/CSI_Control_BIO/PR Controller_0_ref 1/Steper6 ==
  In1 : Inport
  Product : Product
  Step : Step  Time=st_time  SampleTime=0
  Out1 : Outport
  wires:
  Product/1 -> Out1/1
  In1/1 -> Product/1
  Step/1 -> Product/2

== system FDI_sbox_ttime/CSI_Control_Diesel/PR Controller_0_ref 1/Steper6 ==
  In1 : Inport
  Product : Product
  Step : Step  Time=st_time  SampleTime=0
  Out1 : Outport
  wires:
  Product/1 -> Out1/1
  In1/1 -> Product/1
  Step/1 -> Product/2

== matlab function FDI_sbox_ttime/CSI_Control_Diesel/PQ2Iab_PH1 ==
  data: Va input; Ia output; Vb input; p input; q input; Ib output
function [Ia, Ib] = fcn(Va, Vb, p, q)
%#codegen

% divide by zero protection
if(abs((Va^2+Vb^2))<=1000*eps(0))
    det = 1/eps(0);
else
    det = 1/(Va^2+Vb^2); % constante auxiliar
end;
%det = 1/(Va^2+Vb^2);

Mat = det*[Va Vb; Vb -Va];
Iab = Mat*[2*p;2*q];

Iaaux = Iab(1);
Ibaux = Iab(2);

ilim=1e3;

if(Iaaux>ilim)
    Iaaux=ilim;
end;
if(Iaaux<-ilim)
    Iaaux =-ilim;    
end;

if(isnan(Iaaux))
    Iaaux=0;
end;
%-----------------


if(Ibaux>ilim)
    Ibaux=ilim;
end;
if(Ibaux<-ilim)
    Ibaux =-ilim;    
end;

if(isnan(Ibaux))
    Ibaux=0;
end;
%-----------------


Ia = Iaaux;
Ib = Ibaux;

== matlab function FDI_sbox_ttime/CSI_Control_Diesel/PQ_singlePhase ==
  data: va input; p output; vb input; ia input; ib input; q output
function [p, q] = fcn(va, vb, ia, ib)
% Esta funcion calcula la potencia activa y reactiva instantanea
% para el caso mnosofasico. En la revision de 2 papers he observado
% que una manera de extender la teoria de potencia al caso monofasico
% es asumiendo la tension o corriente de una fase como la componente
% alpha y hacer un desfase de 90 grados para obtener una version
% artificial de beta.

paux=va*ia+vb*ib;
if(paux > 20e4)
    paux = 20e4;
end
if(paux < -20e4)
    paux = -20e-4;
end

p = paux/2; % potencia activa instantanea

qaux = vb*ia-va*ib;

if(qaux>20e4)
    qaux=20e4;
end
if(qaux<-20e4)
    qaux=-20e4;
end

q = qaux/2; % potencia reactiva instantanea

== matlab function FDI_sbox_ttime/CSI_Control_BIO/PQ_singlePhase ==
  data: va input; p output; vb input; ia input; ib input; q output
function [p, q] = fcn(va, vb, ia, ib)
% Esta funcion calcula la potencia activa y reactiva instantanea
% para el caso mnosofasico. En la revision de 2 papers he observado
% que una manera de extender la teoria de potencia al caso monofasico
% es asumiendo la tension o corriente de una fase como la componente
% alpha y hacer un desfase de 90 grados para obtener una version
% artificial de beta.

paux=va*ia+vb*ib;
if(paux > 20e4)
    paux = 20e4;
end
if(paux < -20e4)
    paux = -20e-4;
end

p = paux/2; % potencia activa instantanea

qaux = vb*ia-va*ib;

if(qaux>20e4)
    qaux=20e4;
end
if(qaux<-20e4)
    qaux=-20e4;
end

q = qaux/2; % potencia reactiva instantanea

== matlab function FDI_sbox_ttime/Subsystem/SOC  ==
  data: u input; y output
function y = fcn(u)

y = -0.03536*u+100;

== matlab function FDI_sbox_ttime/CSI_Control_BIO/PQ2Iab_PH1 ==
  data: Va input; Ia output; Vb input; p input; q input; Ib output
function [Ia, Ib] = fcn(Va, Vb, p, q)
%#codegen

% divide by zero protection
if(abs((Va^2+Vb^2))<=1000*eps(0))
    det = 1/eps(0);
else
    det = 1/(Va^2+Vb^2); % constante auxiliar
end;
%det = 1/(Va^2+Vb^2);

Mat = det*[Va Vb; Vb -Va];
Iab = Mat*[2*p;2*q];

Iaaux = Iab(1);
Ibaux = Iab(2);

ilim=1e3;

if(Iaaux>ilim)
    Iaaux=ilim;
end;
if(Iaaux<-ilim)
    Iaaux =-ilim;    
end;

if(isnan(Iaaux))
    Iaaux=0;
end;
%-----------------


if(Ibaux>ilim)
    Ibaux=ilim;
end;
if(Ibaux<-ilim)
    Ibaux =-ilim;    
end;

if(isnan(Ibaux))
    Ibaux=0;
end;
%-----------------


Ia = Iaaux;
Ib = Ibaux;

== matlab function FDI_sbox_ttime/LinearProg Potencia Activa ==
  data: P_load input; Pbo output; P_e_alt input; kb input; kd input; PdMax input; PbMax input; Pdo output
function [Pbo, Pdo] = fcn(P_load, P_e_alt, kb, kd, PdMax, PbMax)%, P_e_alt_min)

% P_load es la potencia que se requiere en la carga.

% P_e_alt es la potencia estimada de generacion de las energias
% alternativas

% kb y kd son los pesos de las funcion de costo.

% las salidas son las potencias optimas para bio y diesel

Pb=0;
Pd=0;

flagDelt = 0;

if(P_e_alt >= P_load)
    flagDelt = 1;
end
   

if(flagDelt==0)
    P_trad = P_load - P_e_alt;
    % flag: variable que indica si tiene sentido evaluar los
    % if's que se encuentran mas adelante. es decir, si flag = 0 
    % despues del primer if entonces NO se le esta pidiendo al sistema
    % mas potencia de la que puede generar y portante el problema de 
    % optimizacion lineal tiene sentido.
    % entonces 
    flag=0;

    if(P_trad>PdMax+PbMax)
        Pd=PdMax;
        Pb=PbMax;
        flag=1;
    end

    % si ambas energias tienen el mismo factor de costo.
    if(kd==kb && flag==0)
        Pb=P_trad/2;
        Pd=P_trad/2;
    end

    % si la energia diesel es mas cara que la biomasa.
    if(kd>kb && flag==0)
        if(P_trad<=PbMax)
            Pb=P_trad;
            Pd=0;
        else
            Pb=PbMax;
            Pd=P_trad-PbMax;
        end
    end

    % si la biomasa es mas cara que la diesel.
    if(kd<kb && flag==0)
        if(P_trad<=PdMax)
            Pd=P_trad;
            Pb=0;
        else
            Pd=PdMax;
            Pb=P_trad-PdMax;
        end
    end
end

Pbo=Pb;
Pdo=Pd;

== matlab function FDI_sbox_ttime/LinearProg Potenica Reactiva ==
  data: Q_load input; Qbo output; Q_e_alt input; kb input; kd input; QdMax input; QbMax input; Qdo output
function [Qbo, Qdo] = fcn(Q_load, Q_e_alt, kb, kd, QdMax, QbMax)

% Q_load es la potencia que se requiere en la carga.

% Q_e_alt es la potencia estimada de generacion de las energias
% alternativas

% kb y kd son los pesos de las funcion de costo.

% las salidas son las potencias optimas para bio y diesel

Qb=0;
Qd=0;

flagDelt = 0;

if(Q_e_alt >= Q_load)
    flagDelt = 1;
end
   

if(flagDelt==0)
    Q_trad = Q_load - Q_e_alt;
    % flag: variable que indica si tiene sentido evaluar los
    % if's que se encuentran mas adelante. es decir, si flag = 0 
    % despues del primer if entonces NO se le esta pidiendo al sistema
    % mas potencia de la que puede generar y portanto el problema de 
    % optimizacion lineal tiene sentido.
    % entonces 
    flag=0;

    if(Q_trad>QdMax+QbMax)
        Qd=QdMax;
        Qb=QbMax;
        flag=1;
    end

    % si ambas energias tienen el mismo factor de costo.
    if(kd==kb && flag==0)
        Qb=Q_trad/2;
        Qd=Q_trad/2;
    end

    % si la energia diesel es mas cara que la biomasa.
    if(kd>kb && flag==0)
        if(Q_trad<=QbMax)
            Qb=Q_trad;
            Qd=0;
        else
            Qb=QbMax;
            Qd=Q_trad-QbMax;
        end
    end

    % si la biomasa es mas cara que la diesel.
    if(kd<kb && flag==0)
        if(Q_trad<=QdMax)
            Qd=Q_trad;
            Qb=0;
        else
            Qd=QdMax;
            Qb=Q_trad-QdMax;
        end
    end
end

Qbo=Qb;
Qdo=Qd;

== matlab function FDI_sbox_ttime/MATLAB Function1 ==
  data: SOC input; MaxP output; MaxQ output
function [MaxP, MaxQ] = fcn(SOC)


%  funcion que calcula la potencia maxima que puede suministrar las fuentes
%  renovables deacuerdo a la cantidad de carga que hay almancenada en la
%  bateria. esta va de 0 a 100%


% estoc valores que aparecen a continuacion se pusieron de manera
% arbitraria. corresponde a una persona con especialidad en la parte de
% potencia electrica determinar el verdadero algoritmo para hallar la
% potencia que deberia suministrar el nodo de energia renovable deacuerdo a
% la carga de la bateria.

MaxP = 0;
MaxQ = 0;

if( SOC >= 90 )
    MaxP = 500;
    MaxQ = 5000;
end

if( SOC <= 90 )
    MaxP = 200;
    MaxQ = 4000;
end

if( SOC <= 70 )
    MaxP = 100;
    MaxQ = 1000;
end

if( SOC <= 60 )
    MaxP = 50;
    MaxQ = 500;
end
